simulink model "gm_sampleModel1407_sub"  (R2023a)
settings: Solver=VariableStepAuto  StartTime=0.0  StopTime=10.0  RelTol=1e-3
settings Model: Creator=user1  LastModifiedBy=user1
settings OptimizationCC: BlockReduction=off  ConditionallyExecuteInputs=off
settings DebuggingCC: InheritedTsInSrcMsg=none

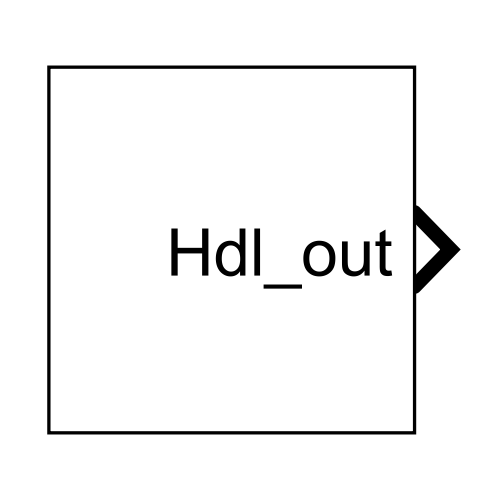
[thumbnail: Simulink's stored preview of the top-level diagram]
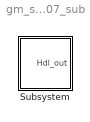
== system gm_sampleModel1407_sub ==
  Subsystem : Subsystem

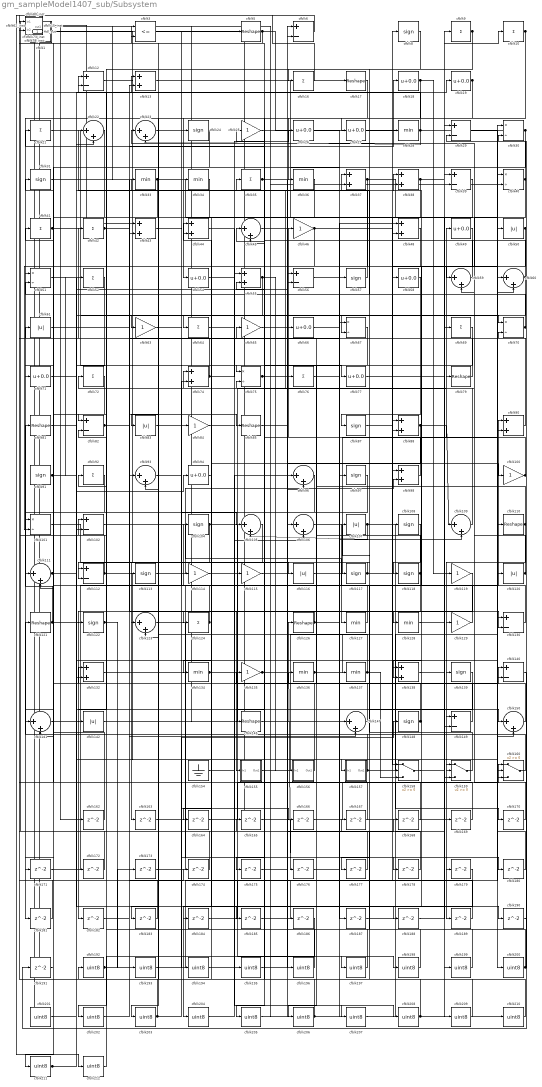
== system gm_sampleModel1407_sub/Subsystem ==
  cfblk1 : Subsystem  mask(Detect Fall Nonpositive){vinit=double(0), InputProcessing=Elements as channels (sample based), OutDataTypeStr=uint8}
      mask prompts: vinit "Simulink:masks:InitialCondition_MP"; InputProcessing "Simulink:masks:InputProcessing_MP"; OutDataTypeStr "Simulink:masks:OutputDataType_MP"
      mask help: Simulink:masks:DetectFallNonpositive_MD
      mask init:
      | InputProcessing = 'Elements as channels (sample based)';
      | OutDataTypeStr = 'uint8';
      | vinit = double(0);
      mask TypeOptions InputProcessing: Simulink:masks:ColumnsAsChannelsFrameBased | Simulink:masks:ElementsAsChannelsSampleBased
      mask TypeOptions OutDataTypeStr: Simulink:masks:uint8 | Simulink:masks:boolean
      mask Display: fprintf('U <= 0\n&  NOT\nU/z <= 0')
  cfblk{9..10,16,21,35,41..42,52,64,69,72,76,92,124} (14 alike) : Sum  Inputs=+  OutDataTypeStr=uint8
  cfblk{25,46,63,65,84,100,114..115,119,129,135} (11 alike) : Gain  OutDataTypeStr=uint8
  cfblk{30,40,51,67,70,75,101} (7 alike) : Product  Inputs=*/  OutDataTypeStr=uint8  RndMeth=Zero  SaturateOnIntegerOverflow=on
  cfblk{6,12,29,39,56,82,102,112,130,140,149} (11 alike) : Sum  Inputs=+-  OutDataTypeStr=uint8
  cfblk{8,24,31,57,87,91,97,104,108,113,117..118,122,139,148} (15 alike) : Signum
  cfblk{22..23,45,59..60,93,96,105..106,109,111,123,141,147,150} (15 alike) : Sum  Inputs=|++  OutDataTypeStr=uint8
  cfblk{50,61,83,107,116,120,142} (7 alike) : Abs  OutDataTypeStr=uint8  SaturateOnIntegerOverflow=off
  cfblk{5,17,79,81,85,110,121,126,145} (9 alike) : Reshape
  cfblk11_inst : Subsystem
  cfblk{28,33..34,36,127..128,134,136..137} (9 alike) : MinMax  OutDataTypeStr=uint8
  cfblk{13,37..38,43..44,48,55,74,88,90,98,132,138} (13 alike) : Sum  OutDataTypeStr=uint8
  cfblk143_inst : Subsystem
  cfblk144_inst : Subsystem
  cfblk14_inst : Subsystem
  cfblk154 : Ground
  cfblk155 : Subsystem
  cfblk156 : Subsystem
  cfblk157 : Subsystem
  cfblk158 : Switch  OutDataTypeStr=uint8  SaturateOnIntegerOverflow=off  InputSameDT=off
  cfblk159 : Switch  OutDataTypeStr=uint8  SaturateOnIntegerOverflow=off  InputSameDT=off
  cfblk15_inst : Subsystem
  cfblk160 : Switch  OutDataTypeStr=uint8  SaturateOnIntegerOverflow=off  InputSameDT=off
  cfblk{162..191} (30 alike) : Delay  SampleTime=1
  cfblk{18..19,26..27,49,54,58,66,71,77,94} (11 alike) : Bias  Bias=0.0  SaturateOnIntegerOverflow=off
  cfblk{192..212} (21 alike) : DataTypeConversion  OutDataTypeStr=uint8  SaturateOnIntegerOverflow=off  RndMeth=Floor
  cfblk2 : Constant  Value=0  OutDataTypeStr=uint8  SampleTime=1
  cfblk3 : RelationalOperator  Operator=<=  OutDataTypeStr=boolean  InputSameDT=off
  cfblk62_inst : Subsystem
  cfblk73_inst : Subsystem
  cfblk78_inst : Subsystem
  cfblk80_inst : Subsystem
  Hdl_out : Outport  OutDataTypeStr=uint8  SampleTime=1
  wires:
  cfblk1/1(Y) -> cfblk75/1, cfblk64/1
  cfblk10/1 -> cfblk27/1, cfblk181/1
  cfblk100/1 -> cfblk49/1, cfblk46/1
  cfblk101/1 -> cfblk116/1
  cfblk102/1 -> cfblk127/1
  cfblk104/1 -> cfblk37/1, cfblk197/1, cfblk112/2
  cfblk105/1 -> cfblk163/1
  cfblk106/1 -> cfblk192/1
  cfblk107/1 -> cfblk105/2, cfblk170/1
  cfblk108/1 -> cfblk118/1
  cfblk109/1 -> cfblk74/1
  cfblk11_inst/1(out1) -> cfblk201/1
  cfblk110/1 -> cfblk66/1, cfblk189/1
  cfblk111/1 -> cfblk149/1, cfblk190/1, cfblk157/1(In1)
  cfblk112/1 -> cfblk159/2, cfblk15_inst/1(in1)
  cfblk113/1 -> cfblk98/2
  cfblk114/1 -> cfblk29/1
  cfblk115/1 -> cfblk128/1
  cfblk116/1 -> cfblk90/1
  cfblk117/1 -> cfblk130/2, cfblk113/1
  cfblk118/1 -> cfblk61/1, cfblk155/1(In1)
  cfblk119/1 -> cfblk182/1
  cfblk12/1 -> cfblk195/1
  cfblk120/1 -> cfblk23/1, cfblk70/2, cfblk72/1
  cfblk121/1 -> cfblk90/2, cfblk81/1
  cfblk122/1 -> cfblk82/2, cfblk193/1
  cfblk123/1 -> cfblk150/1
  cfblk124/1 -> cfblk62_inst/1(in1), cfblk3/1
  cfblk126/1 -> cfblk139/1, cfblk123/1
  cfblk127/1 -> cfblk45/1
  cfblk128/1 -> cfblk9/1
  cfblk129/1 -> cfblk104/1
  cfblk13/1 -> cfblk200/1
  cfblk130/1 -> cfblk38/1
  cfblk132/1 -> cfblk179/1
  cfblk134/1 -> cfblk159/3, cfblk187/1
  cfblk135/1 -> cfblk176/1, cfblk175/1
  cfblk136/1 -> cfblk8/1, cfblk108/1
  cfblk137/1 -> cfblk93/2, cfblk158/3, cfblk25/1
  cfblk138/1 -> cfblk120/1
  cfblk139/1 -> cfblk177/1
  cfblk14_inst/1(out1) -> cfblk91/1
  cfblk140/1 -> cfblk191/1
  cfblk141/1 -> cfblk107/1
  cfblk142/1 -> cfblk79/1
  cfblk143_inst/1(out1) -> cfblk147/1
  cfblk144_inst/1(out1) -> cfblk137/1
  cfblk145/1 -> cfblk196/1
  cfblk147/1 -> cfblk33/1
  cfblk148/1 -> cfblk126/1, cfblk135/1
  cfblk149/1 -> cfblk31/1
  cfblk15_inst/1(out1) -> cfblk40/2, cfblk169/1
  cfblk150/1 -> cfblk76/1
  cfblk154/1 -> cfblk140/1
  cfblk155/1(Out1) -> cfblk98/1
  cfblk156/1(Out1) -> cfblk41/1
  cfblk157/1(Out1) -> cfblk58/1, cfblk55/2, cfblk110/1
  cfblk158/1 -> cfblk39/2
  cfblk159/1 -> cfblk114/1
  cfblk16/1 -> cfblk212/1
  cfblk160/1 -> cfblk121/1
  cfblk162/1 -> cfblk73_inst/1(in1)
  cfblk163/1 -> cfblk48/2
  cfblk164/1 -> cfblk56/2
  cfblk165/1 -> cfblk209/1
  cfblk166/1 -> cfblk149/2
  cfblk167/1 -> cfblk102/1
  cfblk168/1 -> cfblk14_inst/1(in1)
  cfblk169/1 -> cfblk111/1
  cfblk17/1 -> cfblk36/1
  cfblk170/1 -> cfblk59/2
  cfblk171/1 -> cfblk74/2
  cfblk172/1 -> cfblk62_inst/2(in2)
  cfblk173/1 -> cfblk30/1
  cfblk174/1 -> cfblk143_inst/2(in2)
  cfblk175/1 -> cfblk158/2
  cfblk176/1 -> cfblk109/2
  cfblk177/1 -> cfblk45/2
  cfblk178/1 -> cfblk15_inst/2(in2)
  cfblk179/1 -> cfblk204/1
  cfblk18/1 -> cfblk183/1, cfblk119/1
  cfblk180/1 -> cfblk40/1
  cfblk181/1 -> cfblk80_inst/1(in1)
  cfblk182/1 -> cfblk147/2
  cfblk183/1 -> cfblk144_inst/2(in2)
  cfblk184/1 -> cfblk60/1
  cfblk185/1 -> cfblk88/1
  cfblk186/1 -> cfblk202/1
  cfblk187/1 -> cfblk39/1
  cfblk188/1 -> cfblk160/1
  cfblk189/1 -> cfblk11_inst/1(in1)
  cfblk19/1 -> cfblk54/1, cfblk205/1
  cfblk190/1 -> cfblk160/3
  cfblk191/1 -> cfblk1/1(U)
  cfblk192/1 -> cfblk174/1, cfblk173/1
  cfblk193/1 -> cfblk106/1
  cfblk194/1 -> cfblk106/2
  cfblk195/1 -> cfblk168/1
  cfblk196/1 -> cfblk12/1
  cfblk197/1 -> cfblk12/2
  cfblk198/1 -> cfblk167/1
  cfblk199/1 -> cfblk65/1
  cfblk2/1 -> cfblk43/1
  cfblk200/1 -> cfblk30/2, cfblk165/1
  cfblk201/1 -> cfblk13/1
  cfblk202/1 -> cfblk13/2
  cfblk203/1 -> cfblk148/1, cfblk132/1
  cfblk204/1 -> cfblk96/1
  cfblk205/1 -> cfblk96/2
  cfblk206/1 -> cfblk57/1, cfblk123/2
  cfblk207/1 -> cfblk69/1
  cfblk208/1 -> cfblk14_inst/2(in2), cfblk75/2
  cfblk209/1 -> cfblk44/1
  cfblk21/1 -> cfblk77/1
  cfblk210/1 -> cfblk44/2
  cfblk211/1 -> cfblk94/1, cfblk22/2
  cfblk212/1 -> cfblk92/1
  cfblk22/1 -> cfblk71/1
  cfblk23/1 -> cfblk24/1
  cfblk24/1 -> cfblk171/1
  cfblk25/1 -> cfblk97/1
  cfblk26/1 -> cfblk160/2
  cfblk27/1 -> cfblk18/1
  cfblk28/1 -> cfblk78_inst/2(in2), cfblk23/2
  cfblk29/1 -> cfblk50/1
  cfblk3/1 -> cfblk194/1
  cfblk30/1 -> cfblk111/2, Hdl_out/1
  cfblk31/1 -> cfblk129/1
  cfblk33/1 -> cfblk88/2, cfblk43/2
  cfblk34/1 -> cfblk51/1
  cfblk35/1 -> cfblk186/1, cfblk100/1
  cfblk36/1 -> cfblk63/1
  cfblk37/1 -> cfblk83/1, cfblk199/1
  cfblk38/1 -> cfblk184/1, cfblk10/1
  cfblk39/1 -> cfblk142/1
  cfblk40/1 -> cfblk59/1, cfblk29/2
  cfblk41/1 -> cfblk84/1, cfblk67/2
  cfblk42/1 -> cfblk85/1, cfblk28/1
  cfblk43/1 -> cfblk105/1
  cfblk44/1 -> cfblk208/1
  cfblk45/1 -> cfblk6/1
  cfblk46/1 -> cfblk60/2, cfblk101/1
  cfblk48/1 -> cfblk124/1
  cfblk49/1 -> cfblk122/1
  cfblk5/1 -> cfblk73_inst/2(in2), cfblk3/2
  cfblk50/1 -> cfblk188/1, cfblk101/2
  cfblk51/1 -> cfblk172/1
  cfblk52/1 -> cfblk102/2
  cfblk54/1 -> cfblk70/1
  cfblk55/1 -> cfblk132/2, cfblk156/1(In1)
  cfblk56/1 -> cfblk48/1
  cfblk57/1 -> cfblk22/1
  cfblk58/1 -> cfblk117/1
  cfblk59/1 -> cfblk144_inst/1(in1)
  cfblk6/1 -> cfblk143_inst/1(in1)
  cfblk60/1 -> cfblk82/1, cfblk138/2, cfblk185/1, cfblk21/1
  cfblk61/1 -> cfblk93/1
  cfblk62_inst/1(out1) -> cfblk5/1
  cfblk63/1 -> cfblk180/1
  cfblk64/1 -> cfblk26/1
  cfblk65/1 -> cfblk198/1
  cfblk66/1 -> cfblk150/2
  cfblk67/1 -> cfblk145/1
  cfblk69/1 -> cfblk206/1
  cfblk70/1 -> cfblk37/2, cfblk51/2
  cfblk71/1 -> cfblk38/2
  cfblk72/1 -> cfblk141/1
  cfblk73_inst/1(out1) -> cfblk80_inst/2(in2), cfblk34/1
  cfblk74/1 -> cfblk55/1, cfblk207/1, cfblk11_inst/2(in2)
  cfblk75/1 -> cfblk6/2, cfblk159/1
  cfblk76/1 -> cfblk178/1
  cfblk77/1 -> cfblk130/1
  cfblk78_inst/1(out1) -> cfblk17/1
  cfblk79/1 -> cfblk42/1
  cfblk8/1 -> cfblk16/1
  cfblk80_inst/1(out1) -> cfblk210/1, cfblk162/1
  cfblk81/1 -> cfblk56/1
  cfblk82/1 -> cfblk19/1, cfblk67/1
  cfblk83/1 -> cfblk166/1
  cfblk84/1 -> cfblk115/1
  cfblk85/1 -> cfblk136/1
  cfblk87/1 -> cfblk158/1
  cfblk88/1 -> cfblk109/1, cfblk164/1
  cfblk9/1 -> cfblk87/1, cfblk112/1
  cfblk90/1 -> cfblk78_inst/1(in1)
  cfblk91/1 -> cfblk140/2, cfblk52/1
  cfblk92/1 -> cfblk211/1
  cfblk93/1 -> cfblk138/1
  cfblk94/1 -> cfblk134/1
  cfblk96/1 -> cfblk203/1
  cfblk97/1 -> cfblk141/2
  cfblk98/1 -> cfblk35/1

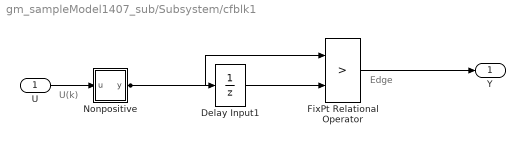
== system gm_sampleModel1407_sub/Subsystem/cfblk1 ==
  note: U(k)
  note: Edge
  U : Inport  OutDataTypeStr=uint8  SampleTime=1
  Delay Input1 : UnitDelay  Description=Store in Global RAM  DisableCoverage=on  InitialCondition=vinit  SampleTime=-1  HasFrameUpgradeWarning=on
  FixPt Relational Operator : RelationalOperator  Operator=>  OutDataTypeStr=fixdt(0, 8)  ZeroCross=off  InputSameDT=off
  Nonpositive : Subsystem  mask(Compare To Zero){relop=<=, OutDataTypeStr=boolean, ZeroCross=off}
      mask prompts: relop "Simulink:masks:Operator_MP"; OutDataTypeStr "Simulink:masks:OutputDataType_MP"; ZeroCross "Simulink:masks:EnableZerocrossingDetection_MP"
      mask help: Simulink:masks:CompareToZero_MD
      mask init:
      | OutDataTypeStr = 'boolean';
      | ZeroCross = 'off';
      | blkName = 'sampleModel1407_sub/Subsystem/cfblk1/Nonpositive';
      | relop = '<=';
      | setValue = 'boolean';
      mask TypeOptions relop: == | ~= | < | <= | >= | >
      mask TypeOptions OutDataTypeStr: Simulink:masks:uint8 | Simulink:masks:boolean
      mask Callback ZeroCross: sl('zeroCrossEnable', gcbh);
      mask Display: disp([relop,' 0'])
  Y : Outport  SampleTime=1
  wires:
  U/1 -> Nonpositive/1(u)
  Delay Input1/1 -> FixPt Relational Operator/2
  FixPt Relational Operator/1 -> Y/1
  Nonpositive/1(y) -> FixPt Relational Operator/1, Delay Input1/1

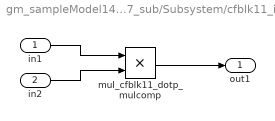
== system gm_sampleModel1407_sub/Subsystem/cfblk11_inst ==
  in1 : Inport  OutDataTypeStr=uint8  SampleTime=1
  in2 : Inport  Port=2  OutDataTypeStr=uint8  SampleTime=1
  mul_cfblk11_dotp_mulcomp : Product  Inputs=**  OutDataTypeStr=uint8  SampleTime=1
  out1 : Outport  OutDataTypeStr=uint8  SampleTime=1
  wires:
  in1/1 -> mul_cfblk11_dotp_mulcomp/1
  in2/1 -> mul_cfblk11_dotp_mulcomp/2
  mul_cfblk11_dotp_mulcomp/1 -> out1/1

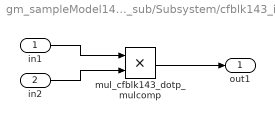
== system gm_sampleModel1407_sub/Subsystem/cfblk143_inst ==
  in1 : Inport  OutDataTypeStr=uint8  SampleTime=1
  in2 : Inport  Port=2  OutDataTypeStr=uint8  SampleTime=1
  mul_cfblk143_dotp_mulcomp : Product  Inputs=**  OutDataTypeStr=uint8  SampleTime=1
  out1 : Outport  OutDataTypeStr=uint8  SampleTime=1
  wires:
  in1/1 -> mul_cfblk143_dotp_mulcomp/1
  in2/1 -> mul_cfblk143_dotp_mulcomp/2
  mul_cfblk143_dotp_mulcomp/1 -> out1/1

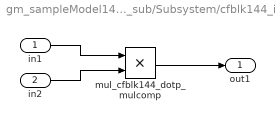
== system gm_sampleModel1407_sub/Subsystem/cfblk144_inst ==
  in1 : Inport  OutDataTypeStr=uint8  SampleTime=1
  in2 : Inport  Port=2  OutDataTypeStr=uint8  SampleTime=1
  mul_cfblk144_dotp_mulcomp : Product  Inputs=**  OutDataTypeStr=uint8  SampleTime=1
  out1 : Outport  OutDataTypeStr=uint8  SampleTime=1
  wires:
  in1/1 -> mul_cfblk144_dotp_mulcomp/1
  in2/1 -> mul_cfblk144_dotp_mulcomp/2
  mul_cfblk144_dotp_mulcomp/1 -> out1/1

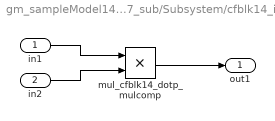
== system gm_sampleModel1407_sub/Subsystem/cfblk14_inst ==
  in1 : Inport  OutDataTypeStr=uint8  SampleTime=1
  in2 : Inport  Port=2  OutDataTypeStr=uint8  SampleTime=1
  mul_cfblk14_dotp_mulcomp : Product  Inputs=**  OutDataTypeStr=uint8  SampleTime=1
  out1 : Outport  OutDataTypeStr=uint8  SampleTime=1
  wires:
  in1/1 -> mul_cfblk14_dotp_mulcomp/1
  in2/1 -> mul_cfblk14_dotp_mulcomp/2
  mul_cfblk14_dotp_mulcomp/1 -> out1/1

== system gm_sampleModel1407_sub/Subsystem/cfblk155 ==
  In1 : Inport  OutDataTypeStr=uint8  PortDimensions=1  SampleTime=1
  Out1 : Outport  SampleTime=1
  wires:
  In1/1 -> Out1/1

== system gm_sampleModel1407_sub/Subsystem/cfblk156 ==
  In1 : Inport  OutDataTypeStr=uint8  PortDimensions=1  SampleTime=1
  Out1 : Outport  SampleTime=1
  wires:
  In1/1 -> Out1/1

== system gm_sampleModel1407_sub/Subsystem/cfblk157 ==
  In1 : Inport  OutDataTypeStr=uint8  PortDimensions=1  SampleTime=1
  Out1 : Outport  SampleTime=1
  wires:
  In1/1 -> Out1/1

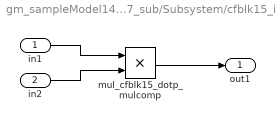
== system gm_sampleModel1407_sub/Subsystem/cfblk15_inst ==
  in1 : Inport  OutDataTypeStr=uint8  SampleTime=1
  in2 : Inport  Port=2  OutDataTypeStr=uint8  SampleTime=1
  mul_cfblk15_dotp_mulcomp : Product  Inputs=**  OutDataTypeStr=uint8  SampleTime=1
  out1 : Outport  OutDataTypeStr=uint8  SampleTime=1
  wires:
  in1/1 -> mul_cfblk15_dotp_mulcomp/1
  in2/1 -> mul_cfblk15_dotp_mulcomp/2
  mul_cfblk15_dotp_mulcomp/1 -> out1/1

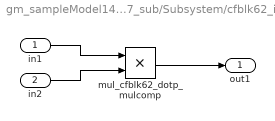
== system gm_sampleModel1407_sub/Subsystem/cfblk62_inst ==
  in1 : Inport  OutDataTypeStr=uint8  SampleTime=1
  in2 : Inport  Port=2  OutDataTypeStr=uint8  SampleTime=1
  mul_cfblk62_dotp_mulcomp : Product  Inputs=**  OutDataTypeStr=uint8  SampleTime=1
  out1 : Outport  OutDataTypeStr=uint8  SampleTime=1
  wires:
  in1/1 -> mul_cfblk62_dotp_mulcomp/1
  in2/1 -> mul_cfblk62_dotp_mulcomp/2
  mul_cfblk62_dotp_mulcomp/1 -> out1/1

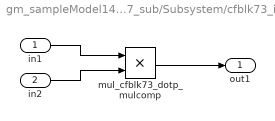
== system gm_sampleModel1407_sub/Subsystem/cfblk73_inst ==
  in1 : Inport  OutDataTypeStr=uint8  SampleTime=1
  in2 : Inport  Port=2  OutDataTypeStr=uint8  SampleTime=1
  mul_cfblk73_dotp_mulcomp : Product  Inputs=**  OutDataTypeStr=uint8  SampleTime=1
  out1 : Outport  OutDataTypeStr=uint8  SampleTime=1
  wires:
  in1/1 -> mul_cfblk73_dotp_mulcomp/1
  in2/1 -> mul_cfblk73_dotp_mulcomp/2
  mul_cfblk73_dotp_mulcomp/1 -> out1/1

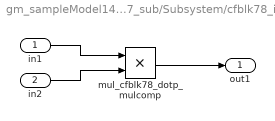
== system gm_sampleModel1407_sub/Subsystem/cfblk78_inst ==
  in1 : Inport  OutDataTypeStr=uint8  SampleTime=1
  in2 : Inport  Port=2  OutDataTypeStr=uint8  SampleTime=1
  mul_cfblk78_dotp_mulcomp : Product  Inputs=**  OutDataTypeStr=uint8  SampleTime=1
  out1 : Outport  OutDataTypeStr=uint8  SampleTime=1
  wires:
  in1/1 -> mul_cfblk78_dotp_mulcomp/1
  in2/1 -> mul_cfblk78_dotp_mulcomp/2
  mul_cfblk78_dotp_mulcomp/1 -> out1/1

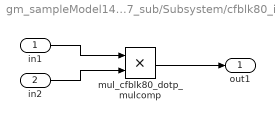
== system gm_sampleModel1407_sub/Subsystem/cfblk80_inst ==
  in1 : Inport  OutDataTypeStr=uint8  SampleTime=1
  in2 : Inport  Port=2  OutDataTypeStr=uint8  SampleTime=1
  mul_cfblk80_dotp_mulcomp : Product  Inputs=**  OutDataTypeStr=uint8  SampleTime=1
  out1 : Outport  OutDataTypeStr=uint8  SampleTime=1
  wires:
  in1/1 -> mul_cfblk80_dotp_mulcomp/1
  in2/1 -> mul_cfblk80_dotp_mulcomp/2
  mul_cfblk80_dotp_mulcomp/1 -> out1/1

== system gm_sampleModel1407_sub/Subsystem/cfblk1/Nonpositive ==
  u : Inport  OutDataTypeStr=uint8  SampleTime=1
  Compare : RelationalOperator  Operator=<=  OutDataTypeStr=boolean  ZeroCross=off
  Constant : Constant  DisableCoverage=on  Value=0  OutDataTypeStr=Inherit: Inherit via back propagation  SampleTime=-1  PreserveConstantTs=on
  y : Outport  SampleTime=1
  wires:
  u/1 -> Compare/1
  Compare/1 -> y/1
  Constant/1 -> Compare/2
